simulink model "laba4_GMSK"  (Simulink 7.5)
settings: Solver=ode45  StartTime=0.0  StopTime=10.0  RelTol=1e-3
undefined symbols (not defined in the file): Fs, get, sided, Two
libraries: dspbuff3 x8, commdigbbndcpm2 x7, commsink2 x4, dspsnks4 x3, commfilt2 x1, commrandsrc2 x1, commutil2 x1
settings Model: Creator=Lenovo  LastModifiedBy=Lenovo

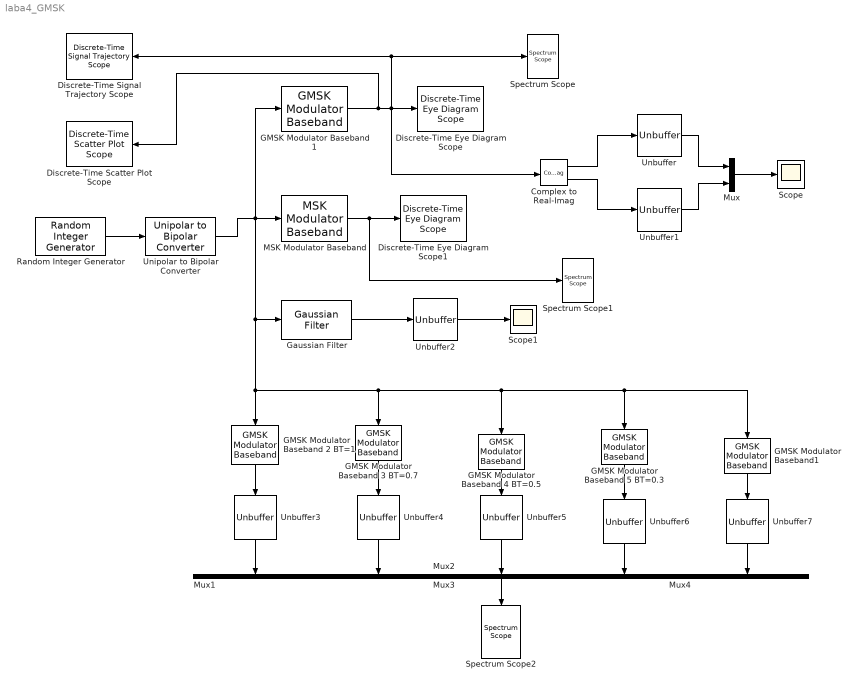
== system laba4_GMSK ==
  Complex to Real-Imag : ComplexToRealImag
  Discrete-Time Eye Diagram Scope : commsink2/Discrete-Time Eye Diagram Scope  Tag=EyeDiagram  SystemSampleTime=-1  sampPerSymb=8  offsetEye=0  symbPerTrace=1  numTraces=40  numNewFrames=10  LineStyles=-  LineColors=b  dupPoints=on  fading=on  render=on  AxisGrid=on  yMin=-3.15  yMax=3.15  inphaseLabel=In-phase Amplitude  quadratureLabel=Quadrature Amplitude  openScopeAtSimStart=on  dispDiagram=In-phase and Quadrature  FrameNumber=off  FigPos=get(0,'defaultfigureposition');  figTitle=Eye Diagram  block_type_=eye  numLinesMax=8
  Discrete-Time Eye Diagram Scope1 : commsink2/Discrete-Time Eye Diagram Scope  Tag=EyeDiagram  SystemSampleTime=-1  sampPerSymb=8  offsetEye=0  symbPerTrace=1  numTraces=40  numNewFrames=10  LineStyles=-  LineColors=b  dupPoints=on  fading=on  render=on  AxisGrid=on  yMin=-3.15  yMax=3.15  inphaseLabel=In-phase Amplitude  quadratureLabel=Quadrature Amplitude  openScopeAtSimStart=on  dispDiagram=In-phase and Quadrature  FrameNumber=off  FigPos=get(0,'defaultfigureposition');  figTitle=Eye Diagram  block_type_=eye  numLinesMax=8
  Discrete-Time Scatter Plot Scope : commsink2/Discrete-Time Scatter Plot Scope  Tag=ScatterPlot  SystemSampleTime=-1  sampPerSymb=1  offsetEye=0  numTraces=40  numNewFrames=10  LineMarkers=.  LineColors=b  fading=on  render=on  AxisGrid=on  xMin=-3.3  xMax=3.315  yMin=-3.3  yMax=3.315  inphaseLabel=In-phase Amplitude  quadratureLabel=Quadrature Amplitude  openScopeAtSimStart=on  FrameNumber=off  FigPos=get(0,'defaultfigureposition');  figTitle=Scatter Plot  numLinesMax=8  block_type_=scatter
  Discrete-Time Signal Trajectory Scope : commsink2/Discrete-Time Signal Trajectory Scope  Tag=SignalTrajectory  SystemSampleTime=-1  sampPerSymb=8  offsetEye=0  numTraces=40  numNewFrames=10  LineStyles=-  LineColors=b  fading=on  render=on  AxisGrid=on  xMin=-3.3  xMax=3.315  yMin=-3.3  yMax=3.315  inphaseLabel=In-phase Amplitude  quadratureLabel=Quadrature Amplitude  openScopeAtSimStart=on  FrameNumber=off  FigPos=get(0,'defaultfigureposition');  figTitle=Signal Trajectory  numLinesMax=8  block_type_=xy
  GMSK Modulator Baseband 1 : commdigbbndcpm2/GMSK Modulator Baseband  SystemSampleTime=-1  inputType=Integer  BT=.3  pulseLength=4  preHistory=1  phaseOffset=0  samplesPerSymbol=8  outDataType=double
  GMSK Modulator Baseband 2 BT=1 : commdigbbndcpm2/GMSK Modulator Baseband  SystemSampleTime=-1  inputType=Integer  BT=.3  pulseLength=4  preHistory=1  phaseOffset=0  samplesPerSymbol=8  outDataType=double
  GMSK Modulator Baseband 3 BT=0.7 : commdigbbndcpm2/GMSK Modulator Baseband  SystemSampleTime=-1  inputType=Integer  BT=.3  pulseLength=4  preHistory=1  phaseOffset=0  samplesPerSymbol=8  outDataType=double
  GMSK Modulator Baseband 4 BT=0.5 : commdigbbndcpm2/GMSK Modulator Baseband  SystemSampleTime=-1  inputType=Integer  BT=.3  pulseLength=4  preHistory=1  phaseOffset=0  samplesPerSymbol=8  outDataType=double
  GMSK Modulator Baseband 5 BT=0.3 : commdigbbndcpm2/GMSK Modulator Baseband  SystemSampleTime=-1  inputType=Integer  BT=.3  pulseLength=4  preHistory=1  phaseOffset=0  samplesPerSymbol=8  outDataType=double
  GMSK Modulator Baseband1 : commdigbbndcpm2/GMSK Modulator Baseband  SystemSampleTime=-1  inputType=Integer  BT=.3  pulseLength=4  preHistory=1  phaseOffset=0  samplesPerSymbol=8  outDataType=double
  Gaussian Filter : commfilt2/Gaussian Filter  DialogController=dspDDGCreate  DialogControllerArgs=DataTag0  SystemSampleTime=-1  N=8  BT=0.3  D=2  sampMode=Frame-based  normMode=Sum of coefficients  filterGain=1  checkCoeff=off  variableName=gaussFilt  launchFVT=off  roundingMode=Floor  overflowMode=off
  MSK Modulator Baseband : commdigbbndcpm2/MSK Modulator Baseband  SystemSampleTime=-1  inputType=Integer  phaseOffset=0  samplesPerSymbol=8  outDataType=double
  Mux{,2..4} (4 alike) : Mux  Inputs=2
  Mux1 : Mux  Inputs=5
  Random Integer Generator : commrandsrc2/Random Integer Generator  SystemSampleTime=-1  mul=2  seed=500  Ts=1/270000  frameBased=on  sampPerFrame=1  orient=off  outDataType=uint32
  Scope : Scope
  Scope1 : Scope
  Spectrum Scope : dspsnks4/Spectrum Scope  DialogController=dspdialog.SpectrumScope  DialogControllerArgs=DataTag1  SystemSampleTime=-1  ScopeProperties=on  Domain=Frequency  HorizSpan=1  UseBuffer=on  BufferSize=128  Overlap=0  inpFftLenInherit=off  FFTlength=128  numAvg=2  DisplayProperties=off  AxisGrid=on  Memory=off  FrameNumber=on  AxisLegend=off  AxisZoom=off  OpenScopeAtSimStart=on  OpenScopeImmediately=off  FigPos=get(0,'defaultfigureposition')  AxisProperties=off  XUnits=Hertz  XRange=Two-sided ((-Fs/2...Fs/2])  XDisplay=0  InheritXIncr=on  XIncr=1.0  XLabel=Samples  XLimit=Auto  YUnits=dBW/Hertz  XMax=1  XMin=0  YLabel=Magnitude-squared, dB  LineProperties=off  wintypeSpecScope=Hann  RsSpecScope=50  betaSpecScope=5  winsampSpecScope=Periodic  XAxisParamsVer=6.9
      settings: YMin=-10  YMax=10
  Spectrum Scope1 : dspsnks4/Spectrum Scope  DialogController=dspdialog.SpectrumScope  DialogControllerArgs=DataTag2  SystemSampleTime=-1  ScopeProperties=on  Domain=Frequency  HorizSpan=1  UseBuffer=off  BufferSize=128  Overlap=64  inpFftLenInherit=off  FFTlength=128  numAvg=2  DisplayProperties=off  AxisGrid=on  Memory=off  FrameNumber=on  AxisLegend=off  AxisZoom=off  OpenScopeAtSimStart=on  OpenScopeImmediately=off  FigPos=get(0,'defaultfigureposition')  AxisProperties=off  XUnits=Hertz  XRange=Two-sided ((-Fs/2...Fs/2])  XDisplay=0  InheritXIncr=on  XIncr=1.0  XLabel=Samples  XLimit=Auto  YUnits=dBW/Hertz  XMax=1  XMin=0  YLabel=Magnitude-squared, dB  LineProperties=off  wintypeSpecScope=Hann  RsSpecScope=50  betaSpecScope=5  winsampSpecScope=Periodic  XAxisParamsVer=6.9
      settings: YMin=-10  YMax=10
  Spectrum Scope2 : dspsnks4/Spectrum Scope  DialogController=dspdialog.SpectrumScope  DialogControllerArgs=DataTag3  SystemSampleTime=-1  ScopeProperties=on  Domain=Frequency  HorizSpan=1  UseBuffer=off  BufferSize=128  Overlap=64  inpFftLenInherit=off  FFTlength=128  numAvg=2  DisplayProperties=off  AxisGrid=on  Memory=off  FrameNumber=on  AxisLegend=off  AxisZoom=off  OpenScopeAtSimStart=on  OpenScopeImmediately=off  FigPos=get(0,'defaultfigureposition')  AxisProperties=off  XUnits=Hertz  XRange=Two-sided ((-Fs/2...Fs/2])  XDisplay=0  InheritXIncr=on  XIncr=1.0  XLabel=Samples  XLimit=Auto  YUnits=dBW/Hertz  XMax=1  XMin=0  YLabel=Magnitude-squared, dB  LineProperties=off  wintypeSpecScope=Hann  RsSpecScope=50  betaSpecScope=5  winsampSpecScope=Periodic  XAxisParamsVer=6.9
      settings: YMin=-10  YMax=10
  Unbuffer{,1..7} (8 alike) : dspbuff3/Unbuffer  ic=0
  Unipolar to Bipolar Converter : commutil2/Unipolar to Bipolar Converter  SystemSampleTime=-1  M=2  polarity=Positive  dataType=double
  wires:
  Random Integer Generator/1 -> Unipolar to Bipolar Converter/1
  Unipolar to Bipolar Converter/1 -> MSK Modulator Baseband/1, GMSK Modulator Baseband 1/1, Gaussian Filter/1, GMSK Modulator Baseband 2 BT=1/1, GMSK Modulator Baseband 3 BT=0.7/1, GMSK Modulator Baseband 4 BT=0.5/1, GMSK Modulator Baseband 5 BT=0.3/1, GMSK Modulator Baseband1/1
  GMSK Modulator Baseband 2 BT=1/1 -> Unbuffer3/1
  GMSK Modulator Baseband 3 BT=0.7/1 -> Unbuffer4/1
  GMSK Modulator Baseband1/1 -> Unbuffer7/1
  GMSK Modulator Baseband 5 BT=0.3/1 -> Unbuffer6/1
  GMSK Modulator Baseband 4 BT=0.5/1 -> Unbuffer5/1
  Unbuffer3/1 -> Mux1/1
  Unbuffer4/1 -> Mux1/2
  Unbuffer5/1 -> Mux1/3
  Unbuffer6/1 -> Mux1/4
  Unbuffer7/1 -> Mux1/5
  Mux1/1 -> Spectrum Scope2/1
  GMSK Modulator Baseband 1/1 -> Discrete-Time Scatter Plot Scope/1, Discrete-Time Eye Diagram Scope/1, Complex to Real-Imag/1, Discrete-Time Signal Trajectory Scope/1, Spectrum Scope/1
  Complex to Real-Imag/1 -> Unbuffer/1
  Complex to Real-Imag/2 -> Unbuffer1/1
  Unbuffer/1 -> Mux/1
  Unbuffer1/1 -> Mux/2
  Mux/1 -> Scope/1
  MSK Modulator Baseband/1 -> Discrete-Time Eye Diagram Scope1/1, Spectrum Scope1/1
  Gaussian Filter/1 -> Unbuffer2/1
  Unbuffer2/1 -> Scope1/1
